simulink model "LL_rdf2"  (R2015b)
settings: Solver=ode45  StartTime=0.0  StopTime=15  MaxStep=1/400  RelTol=1e-3
undefined symbols (not defined in the file): j, LO_Noise_1, LO_Noise_2
libraries: simulink x4, simulink_extras x3
settings Model: Creator=rmg37  LastModifiedBy=gkeating
settings DataIOCC: SaveFormat=Array
settings DebuggingCC: UnderspecifiedInitializationDetection=Classic  MergeDetectMultiDrivingBlocksExec=none  SolverPrmCheckMsg=warning  MultiTaskDSMMsg=warning  MultiTaskCondExecSysMsg=none  FcnCallInpInsideContextMsg=EnableAllAsWarning
settings HardwareCC: ProdBitPerPointer=32  ProdLargestAtomicFloat=None  ProdIntDivRoundTo=Undefined  ProdEndianess=Unspecified  ProdWordSize=32  ProdHWDeviceType=32-bit Generic
settings GRTTargetCC: GeneratePreprocessorConditionals=Disable all
settings ConfigComp: CovModelRefEnable=Off

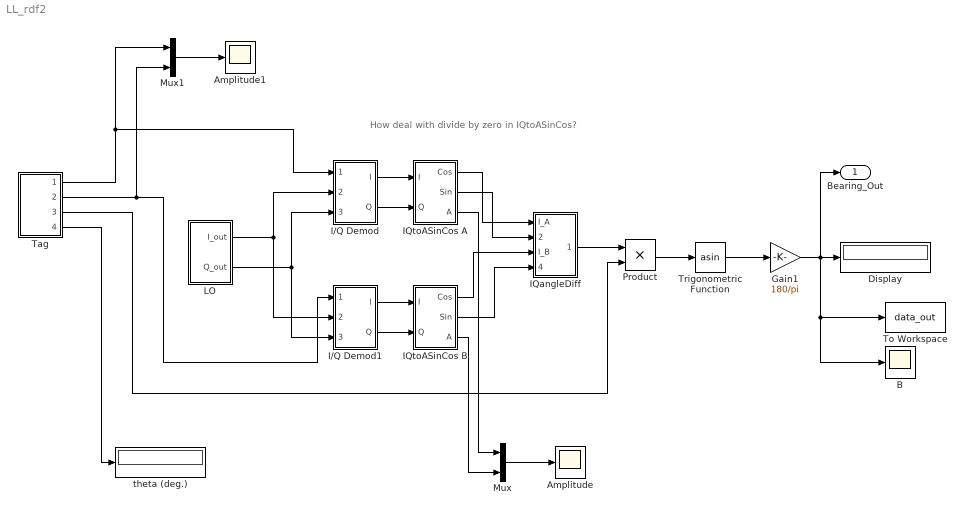
== system LL_rdf2 ==
  note: How deal with divide by zero in IQtoASinCos?
  Amplitude : Scope
  Amplitude1 : Scope
  "B " : Scope
  Display : Display
  Gain1 : Gain  Gain=180/pi
  I/Q Demod : Subsystem
  I/Q Demod1 : Subsystem
  IQangleDiff : Subsystem
  "IQtoASinCos A " : Subsystem
  IQtoASinCos B : Subsystem
  LO : Subsystem  mask{noise_i=LO_Noise_1(j), noise_q=LO_Noise_2(j)}
      mask prompts: noise_i "Noise Level (I)"; noise_q "Noise Level (Q)"
  Mux : Mux  Inputs=2
  Mux1 : Mux  Inputs=2
  Product : Product
  Tag : Subsystem  mask(Angle of Arrival){sep=0.45, off_angle_deg=45, np_1=1e-06, np_2=1e-06}
      mask prompts: sep "Separation (wavelengths)"; off_angle_deg "Off angle (degrees)"; np_1 "Noise Power 1"; np_2 "Noise Power 2"
      mask help: Simulates the angle of arrival of a signal at a phased array
      mask Display:
      | port_label('output', 1, 'RF 1')
      | port_label('output', 2, 'RF 2')
      | port_label('output', 3, 'd/lam')
      | port_label('output', 4, 'theta')
  To Workspace : ToWorkspace  VariableName=data_out  SaveFormat=Structure With Time  SampleTime=-1
      settings: Decimation=3
  Trigonometric Function : Trigonometry  Operator=asin
  "theta (deg.) " : Display
  Bearing_Out : Outport
  wires:
  I/Q Demod/1(I) -> "IQtoASinCos A "/1(I)
  I/Q Demod/2(Q) -> "IQtoASinCos A "/2(Q)
  I/Q Demod1/1(I) -> IQtoASinCos B/1(I)
  I/Q Demod1/2(Q) -> IQtoASinCos B/2(Q)
  Mux/1 -> Amplitude/1
  "IQtoASinCos A "/3(A) -> Mux/1
  IQtoASinCos B/3(A) -> Mux/2
  IQangleDiff/1(A-B) -> Product/1
  "IQtoASinCos A "/1(Cos) -> IQangleDiff/1(I_A)
  "IQtoASinCos A "/2(Sin) -> IQangleDiff/2(Q_A)
  IQtoASinCos B/1(Cos) -> IQangleDiff/3(I_B)
  IQtoASinCos B/2(Sin) -> IQangleDiff/4(Q_B)
  Tag/1(ANT_1) -> I/Q Demod/1(RF in), Mux1/1
  Tag/2(ANT_2) -> Mux1/2, I/Q Demod1/1(RF in)
  Gain1/1 -> To Workspace/1, "B "/1, Display/1, Bearing_Out/1
  Product/1 -> Trigonometric Function/1
  Trigonometric Function/1 -> Gain1/1
  Tag/3(Distance) -> Product/2
  Tag/4("Bearing ") -> "theta (deg.) "/1
  Mux1/1 -> Amplitude1/1
  LO/1("I_out ") -> I/Q Demod/2(LO_I), I/Q Demod1/2(LO_I)
  LO/2("Q_out ") -> I/Q Demod1/3("LO_Q "), I/Q Demod/3("LO_Q ")

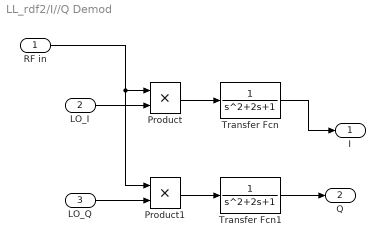
== system LL_rdf2/I//Q Demod ==
  RF in : Inport
  LO_I : Inport  Port=2
  "LO_Q " : Inport  Port=3
  Product : Product
  Product1 : Product
  Transfer Fcn : TransferFcn
  Transfer Fcn1 : TransferFcn
  I : Outport
  Q : Outport  Port=2
  wires:
  LO_I/1 -> Product/2
  Product/1 -> Transfer Fcn/1
  Transfer Fcn/1 -> I/1
  "LO_Q "/1 -> Product1/2
  Product1/1 -> Transfer Fcn1/1
  Transfer Fcn1/1 -> Q/1
  RF in/1 -> Product1/1, Product/1

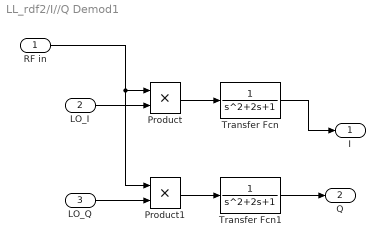
== system LL_rdf2/I//Q Demod1 ==
  RF in : Inport
  LO_I : Inport  Port=2
  "LO_Q " : Inport  Port=3
  Product : Product
  Product1 : Product
  Transfer Fcn : TransferFcn
  Transfer Fcn1 : TransferFcn
  I : Outport
  Q : Outport  Port=2
  wires:
  LO_I/1 -> Product/2
  Product/1 -> Transfer Fcn/1
  Transfer Fcn/1 -> I/1
  "LO_Q "/1 -> Product1/2
  Product1/1 -> Transfer Fcn1/1
  Transfer Fcn1/1 -> Q/1
  RF in/1 -> Product1/1, Product/1

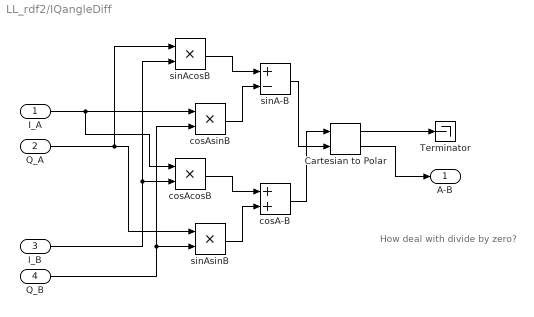
== system LL_rdf2/IQangleDiff ==
  note: How deal with divide by zero?
  I_A : Inport
  Q_A : Inport  Port=2
  I_B : Inport  Port=3
  Q_B : Inport  Port=4
  Cartesian to Polar : simulink_extras/Transformations/Cartesian to Polar
  Terminator : Terminator
  cosA-B : Sum
  cosAcosB : Product
  cosAsinB : Product
  sinA-B : Sum  Inputs=+-
  sinAcosB : Product
  sinAsinB : Product
  A-B : Outport
  wires:
  I_B/1 -> sinAcosB/2, cosAcosB/2
  sinAcosB/1 -> sinA-B/1
  sinA-B/1 -> Cartesian to Polar/2
  sinAsinB/1 -> cosA-B/2
  Q_A/1 -> sinAsinB/1, sinAcosB/1
  cosA-B/1 -> Cartesian to Polar/1
  I_A/1 -> cosAcosB/1, cosAsinB/1
  Cartesian to Polar/1 -> Terminator/1
  Q_B/1 -> sinAsinB/2, cosAsinB/2
  Cartesian to Polar/2 -> A-B/1
  cosAsinB/1 -> sinA-B/2
  cosAcosB/1 -> cosA-B/1

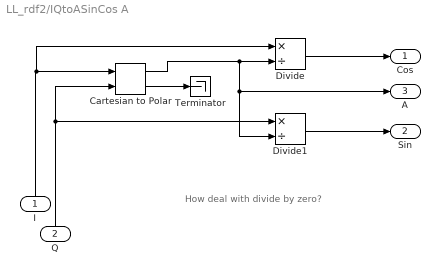
== system LL_rdf2/IQtoASinCos A  ==
  note: How deal with divide by zero?
  I : Inport
  Q : Inport  Port=2
  Cartesian to Polar : simulink_extras/Transformations/Cartesian to Polar
  Divide : Product  Inputs=*/
  Divide1 : Product  Inputs=*/
  Terminator : Terminator
  Cos : Outport
  Sin : Outport  Port=2
  A : Outport  Port=3
  wires:
  Divide1/1 -> Sin/1
  Cartesian to Polar/2 -> Terminator/1
  Divide/1 -> Cos/1
  I/1 -> Divide/1, Cartesian to Polar/1
  Cartesian to Polar/1 -> A/1, Divide1/2, Divide/2
  Q/1 -> Cartesian to Polar/2, Divide1/1

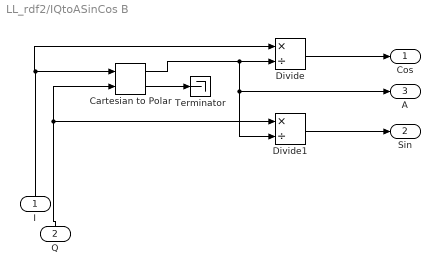
== system LL_rdf2/IQtoASinCos B ==
  I : Inport
  Q : Inport  Port=2
  Cartesian to Polar : simulink_extras/Transformations/Cartesian to Polar
  Divide : Product  Inputs=*/
  Divide1 : Product  Inputs=*/
  Terminator : Terminator
  Cos : Outport
  Sin : Outport  Port=2
  A : Outport  Port=3
  wires:
  Divide1/1 -> Sin/1
  Cartesian to Polar/2 -> Terminator/1
  Divide/1 -> Cos/1
  I/1 -> Divide/1, Cartesian to Polar/1
  Cartesian to Polar/1 -> A/1, Divide1/2, Divide/2
  Q/1 -> Cartesian to Polar/2, Divide1/1

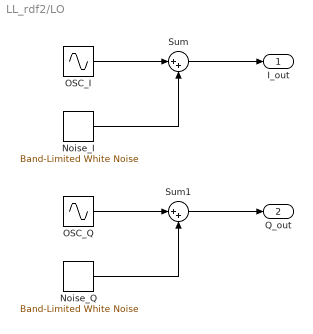
== system LL_rdf2/LO ==
  Noise_I : simulink/Sources/Band-Limited White Noise  Cov=noise_i  Ts=.001  seed=[23341]
  Noise_Q : simulink/Sources/Band-Limited White Noise  Cov=1e-5  Ts=.001  seed=[23341]
  "OSC_I " : Sin  Frequency=2*pi*100  SampleTime=0
  OSC_Q : Sin  Frequency=2*pi*100  Phase=pi/2  SampleTime=0
  Sum : Sum  Inputs=|++
  Sum1 : Sum  Inputs=|++
  "I_out " : Outport
  "Q_out " : Outport  Port=2
  wires:
  Noise_I/1 -> Sum/2
  "OSC_I "/1 -> Sum/1
  Sum/1 -> "I_out "/1
  Noise_Q/1 -> Sum1/2
  OSC_Q/1 -> Sum1/1
  Sum1/1 -> "Q_out "/1

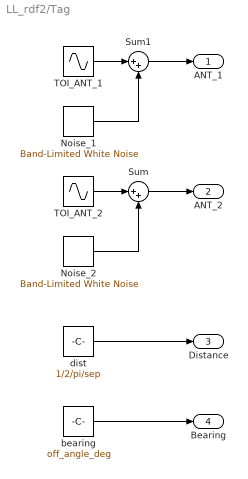
== system LL_rdf2/Tag ==
  Noise_1 : simulink/Sources/Band-Limited White Noise  Cov=np_1  Ts=0.001  seed=462
  Noise_2 : simulink/Sources/Band-Limited White Noise  Cov=np_2  Ts=.001  seed=462
  Sum : Sum  Inputs=|++
  Sum1 : Sum  Inputs=|++
  TOI_ANT_1 : Sin  Frequency=2*pi*99.9  SampleTime=0
  TOI_ANT_2 : Sin  Frequency=2*pi*99.9  Phase=-2*pi*sep*sin(pi*off_angle_deg/180)  SampleTime=0
  bearing : Constant  Value=off_angle_deg
  "dist " : Constant  Value=1/2/pi/sep
  ANT_1 : Outport
  ANT_2 : Outport  Port=2
  Distance : Outport  Port=3
  "Bearing " : Outport  Port=4
  wires:
  "dist "/1 -> Distance/1
  bearing/1 -> "Bearing "/1
  TOI_ANT_1/1 -> Sum1/1
  Noise_1/1 -> Sum1/2
  Sum1/1 -> ANT_1/1
  TOI_ANT_2/1 -> Sum/1
  Noise_2/1 -> Sum/2
  Sum/1 -> ANT_2/1
